simulink model "BoatDynamic"  (R2014a)
settings: Solver=ode3  StartTime=0.0  StopTime=10.0  FixedStep=0.1  RelTol=1e-3
values from neighbouring files (symbols this model uses):
  alphacoeff_xdata = alphacoeff_xdata2    [param.m]
  alphacoeff_yddata = interp1(alphacoeff_xdata,alphacoeff_yddata,alphacoeff_xdata2,'pchip')    [param.m]
  alphacoeff_yldata = interp1(alphacoeff_xdata,alphacoeff_yldata,alphacoeff_xdata2,'pchip')    [param.m]
  hull_xdata = hull_xdata2    [param.m]
  hull_ydata = arrayfun(@(x)resistancehull(x),hull_xdata2)    [param.m]
  keelcoeff_xdata = keelcoeff_xdata2    [param.m]
  keelcoeff_yddata = interp1(keelcoeff_xdata,keelcoeff_yddata,keelcoeff_xdata2,'pchip')    [param.m]
  keelcoeff_yldata = interp1(keelcoeff_xdata,keelcoeff_yldata,keelcoeff_xdata2,'pchip')    [param.m]
  ruddercoeff_xdata = ruddercoeff_xdata2    [param.m]
  ruddercoeff_yddata = arrayfun(@(x)ruddercoef_cdr(x),ruddercoeff_xdata2)    [param.m]
  ruddercoeff_yldata = interp1(ruddercoeff_xdata,ruddercoeff_yldata,ruddercoeff_xdata2,'pchip')    [param.m]
settings Model: Creator=paul  LastModifiedBy=rousse
settings DataIOCC: SaveOutput=off  SaveTime=off
settings HardwareCC: ProdHWDeviceType=Generic->Unspecified (assume 32-bit Generic)
settings RTWCC: GenCodeOnly=on  RTWVerbose=off  ProcessScript=grt_make_rtw_hook
settings GRTTargetCC: MatFileLogging=off

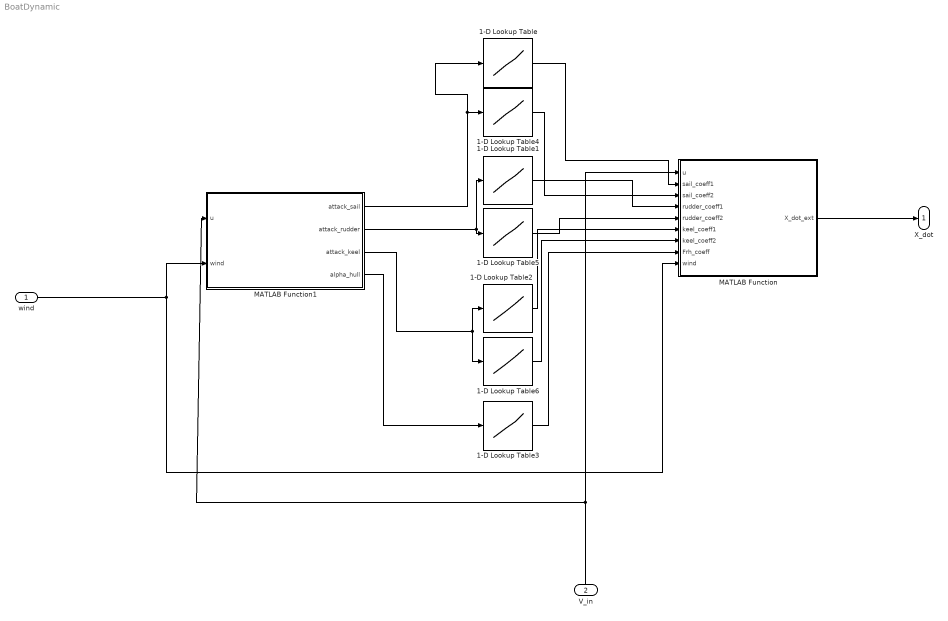
== system BoatDynamic ==
  wind : Inport  PortDimensions=2
  V_in : Inport  Port=2  PortDimensions=12
  1-D Lookup Table : Lookup_n-D  NumberOfTableDimensions=1  BreakpointsForDimension1=alphacoeff_xdata  Table=alphacoeff_yldata  InterpMethod=Cubic spline  RndMeth=Simplest  InputSameDT=on
  1-D Lookup Table1 : Lookup_n-D  NumberOfTableDimensions=1  BreakpointsForDimension1=ruddercoeff_xdata  Table=ruddercoeff_yldata  InterpMethod=Cubic spline  RndMeth=Simplest  InputSameDT=on
  1-D Lookup Table2 : Lookup_n-D  NumberOfTableDimensions=1  BreakpointsForDimension1=keelcoeff_xdata  Table=keelcoeff_yldata  InterpMethod=Cubic spline  DiagnosticForOutOfRangeInput=Warning  RndMeth=Simplest  InputSameDT=on
  1-D Lookup Table3 : Lookup_n-D  NumberOfTableDimensions=1  BreakpointsForDimension1=hull_xdata  Table=hull_ydata  RndMeth=Simplest  InputSameDT=on
  1-D Lookup Table4 : Lookup_n-D  NumberOfTableDimensions=1  BreakpointsForDimension1=alphacoeff_xdata  Table=alphacoeff_yddata  InterpMethod=Cubic spline  RndMeth=Simplest  InputSameDT=on
  1-D Lookup Table5 : Lookup_n-D  NumberOfTableDimensions=1  BreakpointsForDimension1=ruddercoeff_xdata  Table=ruddercoeff_yddata  InterpMethod=Cubic spline  RndMeth=Simplest  InputSameDT=on
  1-D Lookup Table6 : Lookup_n-D  NumberOfTableDimensions=1  BreakpointsForDimension1=keelcoeff_xdata  Table=keelcoeff_yddata  InterpMethod=Cubic spline  RndMeth=Simplest  InputSameDT=on
  MATLAB Function : MATLAB Function  TreatAsAtomicUnit=on
  MATLAB Function1 : MATLAB Function  TreatAsAtomicUnit=on
  X_dot : Outport  PortDimensions=9
  wires:
  1-D Lookup Table4/1 -> MATLAB Function/3(sail_coeff2)
  V_in/1 -> MATLAB Function/1(u), MATLAB Function1/1(u)
  MATLAB Function1/1(attack_sail) -> 1-D Lookup Table/1, 1-D Lookup Table4/1
  MATLAB Function1/4(alpha_hull) -> 1-D Lookup Table3/1
  1-D Lookup Table6/1 -> MATLAB Function/7(keel_coeff2)
  1-D Lookup Table3/1 -> MATLAB Function/8(Frh_coeff)
  1-D Lookup Table2/1 -> MATLAB Function/6(keel_coeff1)
  1-D Lookup Table/1 -> MATLAB Function/2(sail_coeff1)
  MATLAB Function1/2(attack_rudder) -> 1-D Lookup Table1/1, 1-D Lookup Table5/1
  1-D Lookup Table1/1 -> MATLAB Function/4(rudder_coeff1)
  1-D Lookup Table5/1 -> MATLAB Function/5(rudder_coeff2)
  MATLAB Function/1(X_dot_ext) -> X_dot/1
  wind/1 -> MATLAB Function/9(wind), MATLAB Function1/2(wind)
  MATLAB Function1/3(attack_keel) -> 1-D Lookup Table2/1, 1-D Lookup Table6/1

== matlab function BoatDynamic/MATLAB Function1 ==
  data: u input; attack_sail output; attack_rudder output; attack_keel output; alpha_hull output; wind input
% interpreted Matlab function "f.m" for the Simulink file "SailingYachtModel.slx"
% This function describes the dynamics of a 4DOF sailing yacht model
% and gives the derivative of the state X and the sail angle delta_s.
% The input vector V_in contains the system state and the control input vector. 
%
% For the model description, notations, equations and parameters,
% see Xiao and Jouffroy, "Modeling and nonlinear heading control of sailing
% yachts", IEEE Journal of Oceanic Engineering, vol. 39, no. 2., pp. 256-268, 2014.
% 
% Jerome Jouffroy, Jiaxi He and Lin Xiao, 2014.
% University of Southern Denmark.



function [attack_sail,attack_rudder,attack_keel,alpha_hull]=sailcoeff_attack(u,wind)
%#codegen

% use the system parameters
par = modeleBoat();

par.vt = wind(1);                           % the norm of wind velocity
par.alpha_w = wind(2);                      % the direction of wind (coming from the north, ie going south)


V_in = u;
% retrieve the system state from the field input vector "V_in"
x = V_in(5);
y = V_in(6);
phi = V_in(7);
psi = V_in(8);
u = V_in(9);
v = V_in(10);
p = V_in(11);
r = V_in(12);
nu = [ u ; v ; p ; r ];

% retrieve the input signals from the vector "V_in"
delta_r = V_in(1);
delta_sbar = V_in(2);
y_w = V_in(3);
u_s = V_in(4);


% evaluate the matrix M and C in the model
M_RB = [ par.m 0 0 0 ; 0 par.m 0 0 ; 0 0 par.Ixx -par.Ixz ; 0 0 -par.Ixz par.Izz];
C_RB = [0 -par.m*r 0 0 ; par.m*r 0 0 0 ; 0 0 0 0 ; 0 0 0 0];

M_A = [par.a11 0 0 0;0 par.a22 par.a24 par.a26;0 par.a24 par.a44 par.a46;0 par.a26 par.a46 par.a66];
C_A = [0  0 0 -par.a22*nu(2)-par.a24*nu(3)-par.a26*nu(4) ; 0 0 0 par.a11*nu(1) ; 0 0 0 0 ; par.a22*nu(2)+par.a24*nu(3)+par.a26*nu(4) -par.a11*nu(1) 0 0];

M = M_RB + M_A;

% calculate the tau vector, ie forces and moments generated from:
% the sail
v_t = [ par.vt*cos(par.alpha_w); par.vt*sin(par.alpha_w); 0 ];
v_tw = log(abs(par.z_s)*cos(phi)/par.h0)/log(par.h1/par.h0)*v_t;
R1 = [ cos(-psi) -sin(-psi) 0; sin(-psi) cos(-psi) 0; 0 0 1];
R2 = [ 1 0 0 ; 0 cos(-phi) -sin(-phi); 0 sin(-phi) cos(-phi)];
v_tb = R2*R1*v_tw; % wind expressed in the body frame
V_in = [ u ; v ; 0 ];
V_awb = v_tb - V_in - cross([p;0;r],[par.xs;par.ys;par.zs]);
V_awu = V_awb(1);
V_awv = V_awb(2);
alpha_aw = atan2(V_awv,-V_awu);

%% (sail luffing or not)
if alpha_aw-u_s>delta_sbar
    delta_s = delta_sbar;
elseif alpha_aw-u_s<-delta_sbar
    delta_s = -delta_sbar;
else
    delta_s = alpha_aw-u_s;
end
delta_s = delta_s + u_s;

alpha_as = alpha_aw - delta_s;

attack_sail = alpha_as;

% fit the input angle of attack into the interval [-pi,pi]
if attack_sail > pi
    attack_sail = mod(attack_sail+pi,2*pi) - pi;
else
    if attack_sail < -pi
        attack_sail = mod(attack_sail-pi,-2*pi) + pi;
    end
end

%% the rudder
v_aru = -u+r*par.yr;
v_arv = -v-r*par.xr + p*par.zr;
alpha_ar = atan2(v_arv,-v_aru);
alpha_a = alpha_ar-delta_r;

attack_rudder = alpha_a;

% fit the input angle of attack into the interval [-pi,pi]
if attack_rudder > pi
    attack_rudder = mod(attack_rudder+pi,2*pi) - pi;
else
    if attack_rudder < -pi
        attack_rudder = mod(attack_rudder-pi,-2*pi) + pi;
    end
end

%% the keel
v_aku = -u + r*par.yk;
v_akv = -v - r*par.xk+p*par.zk;
alpha_ak = atan2(v_akv,-v_aku);
alpha_e = alpha_ak;

attack_keel = alpha_e;

% fit the input angle of attack into the interval [-pi,pi]
if attack_keel > pi
    attack_keel = mod(attack_keel+pi,2*pi) - pi;
else
    if attack_keel < -pi
        attack_keel = mod(attack_keel-pi,-2*pi) + pi;
    end
end

%% from the hull
v_ahu = -u + r*par.yh;
v_ahv = (-v-r*par.xh + p*par.zh)/cos(phi);
v_ah = sqrt(v_aku^2+v_akv^2);
alpha_ah = atan2(v_ahv,-v_ahu);
alpha_hull = v_ah;

== matlab function BoatDynamic/MATLAB Function ==
  data: u input; X_dot_ext output; sail_coeff1 input; sail_coeff2 input; rudder_coeff1 input; rudder_coeff2 input; keel_coeff1 input; keel_coeff2 input; Frh_coeff input; wind input
% interpreted Matlab function "f.m" for the Simulink file "SailingYachtModel.slx"
% This function describes the dynamics of a 4DOF sailing yacht model
% and gives the derivative of the state X and the sail angle delta_s.
% The input vector V_in contains the system state and the control input vector. 
%
% For the model description, notations, equations and parameters,
% see Xiao and Jouffroy, "Modeling and nonlinear heading control of sailing
% yachts", IEEE Journal of Oceanic Engineering, vol. 39, no. 2., pp. 256-268, 2014.
% 
% Jerome Jouffroy, Jiaxi He and Lin Xiao, 2014.
% University of Southern Denmark.



function X_dot_ext  =fcn(u,sail_coeff1,sail_coeff2,rudder_coeff1,rudder_coeff2,keel_coeff1,keel_coeff2,Frh_coeff,wind)
%#codegen

% use the system parameters
par = modeleBoat();

par.vt = wind(1);                           % the norm of wind velocity
par.alpha_w = wind(2);                      % the direction of wind (coming from the north, ie going south)


V_in = u;
% retrieve the system state from the field input vector "V_in"
x = V_in(5);
y = V_in(6);
phi = V_in(7);
psi = V_in(8);
u = V_in(9);
v = V_in(10);
p = V_in(11);
r = V_in(12);
nu = [ u ; v ; p ; r ];

% retrieve the input signals from the vector "V_in"
delta_r = V_in(1);
delta_sbar = V_in(2);
y_w = V_in(3);
u_s = V_in(4);

% evaluate the matrix M and C in the model
M_RB = [ par.m 0 0 0 ; 0 par.m 0 0 ; 0 0 par.Ixx -par.Ixz ; 0 0 -par.Ixz par.Izz];
C_RB = [0 -par.m*r 0 0 ; par.m*r 0 0 0 ; 0 0 0 0 ; 0 0 0 0];

M_A = [par.a11 0 0 0;0 par.a22 par.a24 par.a26;0 par.a24 par.a44 par.a46;0 par.a26 par.a46 par.a66];
C_A = [0  0 0 -par.a22*nu(2)-par.a24*nu(3)-par.a26*nu(4) ; 0 0 0 par.a11*nu(1) ; 0 0 0 0 ; par.a22*nu(2)+par.a24*nu(3)+par.a26*nu(4) -par.a11*nu(1) 0 0];

M = M_RB + M_A;

% calculate the tau vector, ie forces and moments generated from:
% the sail
v_t = [ par.vt*cos(par.alpha_w); par.vt*sin(par.alpha_w); 0 ];
v_tw = log(abs(par.z_s)*cos(phi)/par.h0)/log(par.h1/par.h0)*v_t;
R1 = [ cos(-psi) -sin(-psi) 0; sin(-psi) cos(-psi) 0; 0 0 1];
R2 = [ 1 0 0 ; 0 cos(-phi) -sin(-phi); 0 sin(-phi) cos(-phi)];
v_tb = R2*R1*v_tw; % wind expressed in the body frame
V_in = [ u ; v ; 0 ];
V_awb = v_tb - V_in - cross([p;0;r],[par.xs;par.ys;par.zs]);
V_awu = V_awb(1);
V_awv = V_awb(2);
alpha_aw = atan2(V_awv,-V_awu);

% (sail luffing or not)
if alpha_aw-u_s>delta_sbar
    delta_s = delta_sbar;
elseif alpha_aw-u_s<-delta_sbar
    delta_s = -delta_sbar;
else
    delta_s = alpha_aw-u_s;
end
delta_s = delta_s + u_s;

alpha_as = alpha_aw - delta_s;

Cls = sail_coeff1;
Cds = sail_coeff2;

Ls = 0.5*par.rho_a*par.As*(V_awu^2+V_awv^2)*Cls;
Ds = 0.5*par.rho_a*par.As*(V_awu^2+V_awv^2)*Cds;

tau_sail = [Ls*sin(alpha_aw)-Ds*cos(alpha_aw); Ls*cos(alpha_aw)+Ds*sin(alpha_aw);-(Ls*cos(alpha_aw)+Ds*sin(alpha_aw))*par.zs; -(Ls*sin(alpha_aw)-Ds*cos(alpha_aw))*par.Xce*sin(delta_s)+(Ls*cos(alpha_aw)+Ds*sin(alpha_aw))*(par.Xm-par.Xce*cos(delta_s))];
Mzs = tau_sail(4);

% the rudder
v_aru = -u+r*par.yr;
v_arv = -v-r*par.xr + p*par.zr;
alpha_ar = atan2(v_arv,-v_aru);
alpha_a = alpha_ar-delta_r;

%[Clr,Cdr] = ruddercoef(alpha_a);
Clr = rudder_coeff1;
Cdr = rudder_coeff2;

Cdr = Cdr+Clr^2*par.Ar/(pi*2*par.zeta_r*par.d_r^2);

Lr = 0.5*par.rho_w*par.Ar*(v_aru^2+v_arv^2)*Clr;
Dr = 0.5*par.rho_w*par.Ar*(v_aru^2+v_arv^2)*Cdr;

tau_rudder = [Lr*sin(alpha_ar)-Dr*cos(alpha_ar); Lr*cos(alpha_ar)+Dr*sin(alpha_ar); -(Lr*cos(alpha_ar)+Dr*sin(alpha_ar))*par.zr; (Lr*cos(alpha_ar)+Dr*sin(alpha_ar))*par.xr];
Mzr = tau_rudder(4);

% the tau vector is finally given by:
tau = tau_sail + tau_rudder;

% calculate the damping forces and moments:
% from the keel
v_aku = -u + r*par.yk;
v_akv = -v - r*par.xk+p*par.zk;
alpha_ak = atan2(v_akv,-v_aku);
alpha_e = alpha_ak;

Clk = keel_coeff1;
Cdk = keel_coeff2;

Cdk = Cdk + Clk^2*par.Ak/(pi*2*par.zeta_k*par.d_k^2);

Lk = 0.5*par.rho_w*par.Ak*(v_aku^2+v_akv^2)*Clk;
Dk = 0.5*par.rho_w*par.Ak*(v_aku^2+v_akv^2)*Cdk;

D_keel = [ -Lk*sin(alpha_ak)+Dk*cos(alpha_ak); -Lk*cos(alpha_ak)-Dk*sin(alpha_ak); -(-Lk*cos(alpha_ak)-Dk*sin(alpha_ak))*par.zk; -(Lk*cos(alpha_ak)+Dk*sin(alpha_ak))*par.xk];

% from the hull
v_ahu = -u + r*par.yh;
v_ahv = (-v-r*par.xh + p*par.zh)/cos(phi);
v_ah = sqrt(v_aku^2+v_akv^2);
alpha_ah = atan2(v_ahv,-v_ahu);

Frh = Frh_coeff;

D_hull = [Frh*cos(alpha_ah);-Frh*sin(alpha_ah)*cos(phi); Frh*sin(alpha_ah)*cos(phi)*par.zh; -Frh*sin(alpha_ah)*cos(phi)*par.xh];

% from heel and yaw
% (compute first eta_dot and thereby phi_dot and psi_dot)
J = [cos(psi) -sin(psi)*cos(phi) 0 0; sin(psi) cos(psi)*cos(phi) 0 0; 0 0 1 0; 0 0 0 cos(phi)];
eta_dot = J*nu;
phi_dot = eta_dot(3);
psi_dot = eta_dot(4);

D_heelandyaw = [0;0;par.c*phi_dot*abs(phi_dot);par.d*psi_dot*abs(psi_dot)*cos(phi)]; 

% compute total damping vector D
D = D_keel + D_hull + D_heelandyaw;

% righting moment plus internal moving mass system (ie transversal weight)
phi_deg = phi*180/pi;
M_xw = -y_w*par.w_c*par.y_bm*cos(phi);
M_zw = -y_w*par.w_c*par.x_c*sin(abs(phi));
G = [ 0 ; 0 ; par.a*phi_deg^2+par.b*phi_deg + M_xw ; M_zw];

% computation of nu_dot
nu_dot = -M\(C_RB*nu+C_A*nu)-M\D-M\G+M\tau; 
 

% output the derivative of the state extended with the sail angle
X_dot_ext = [ eta_dot   ; 
              nu_dot   ;
              delta_s];
